simulink model "double_pendulum_2"  (R2022a)
settings: Solver=FixedStepAuto  StartTime=0.0  StopTime=100  FixedStep=0.001  RelTol=1e-3
libraries: sm_lib x8, fl_lib x8, nesl_utility x8, simulink x6
settings Model: Creator=keonyoung  LastModifiedBy=keonyoung

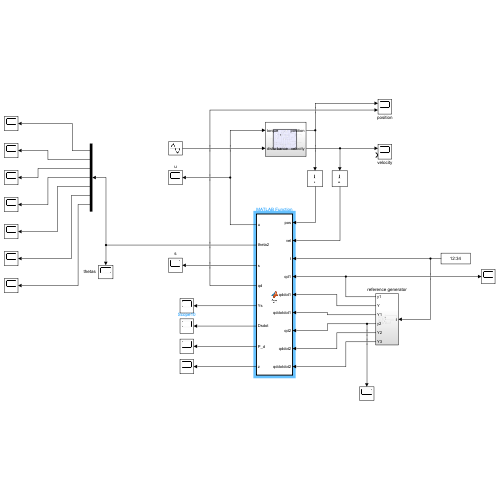
[thumbnail: Simulink's stored preview of the top-level diagram]
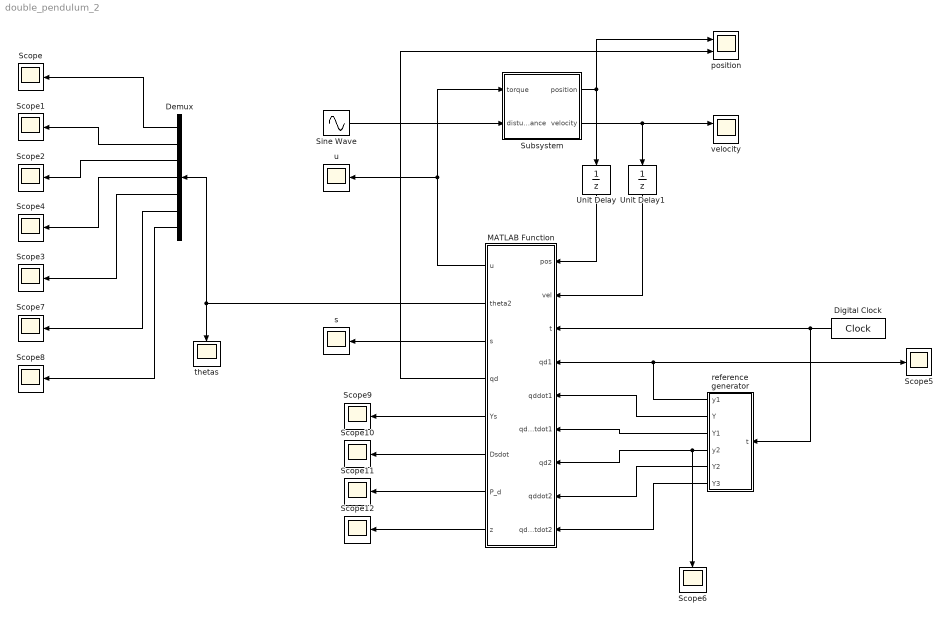
== system double_pendulum_2 ==
  Demux : Demux  Outputs=7
  Digital Clock : DigitalClock  SampleTime=0.001
  MATLAB Function : MATLAB Function  TreatAsAtomicUnit=on
  Scope{,1..12} (13 alike) : Scope
  Sine Wave : Sin  Amplitude=0  SampleTime=0
  Subsystem : Subsystem
  Unit Delay : UnitDelay  SampleTime=-1  HasFrameUpgradeWarning=on
  Unit Delay1 : UnitDelay  SampleTime=-1  HasFrameUpgradeWarning=on
  position : Scope  NumInputPorts=2
  reference generator : Subsystem
  s : Scope
  thetas : Scope
  u : Scope
  velocity : Scope  NumInputPorts=2
  wires:
  MATLAB Function/1(u) -> Subsystem/1(torque), u/1
  Sine Wave/1 -> Subsystem/2(disturbance)
  Subsystem/1(position) -> position/1, Unit Delay/1
  Subsystem/2(velocity) -> Unit Delay1/1, velocity/1
  Digital Clock/1 -> MATLAB Function/3(t), reference generator/1(t)
  Unit Delay/1 -> MATLAB Function/1(pos)
  Unit Delay1/1 -> MATLAB Function/2(vel)
  MATLAB Function/2(theta2) -> Demux/1, thetas/1
  MATLAB Function/3(s) -> s/1
  MATLAB Function/4(qd) -> position/2
  Demux/3 -> Scope2/1
  Demux/4 -> Scope4/1
  Demux/5 -> Scope3/1
  Demux/2 -> Scope1/1
  Demux/1 -> Scope/1
  reference generator/1(y1) -> Scope5/1, MATLAB Function/4(qd1)
  reference generator/2(Y) -> MATLAB Function/5(qddot1)
  reference generator/3(Y1) -> MATLAB Function/6(qddotdot1)
  reference generator/4(y2) -> Scope6/1, MATLAB Function/7(qd2)
  reference generator/5(Y2) -> MATLAB Function/8(qddot2)
  reference generator/6(Y3) -> MATLAB Function/9(qddotdot2)
  Demux/6 -> Scope7/1
  Demux/7 -> Scope8/1
  MATLAB Function/5(Ys) -> Scope9/1
  MATLAB Function/6(Dsdot) -> Scope10/1
  MATLAB Function/7(P_d) -> Scope11/1
  MATLAB Function/8(z) -> Scope12/1

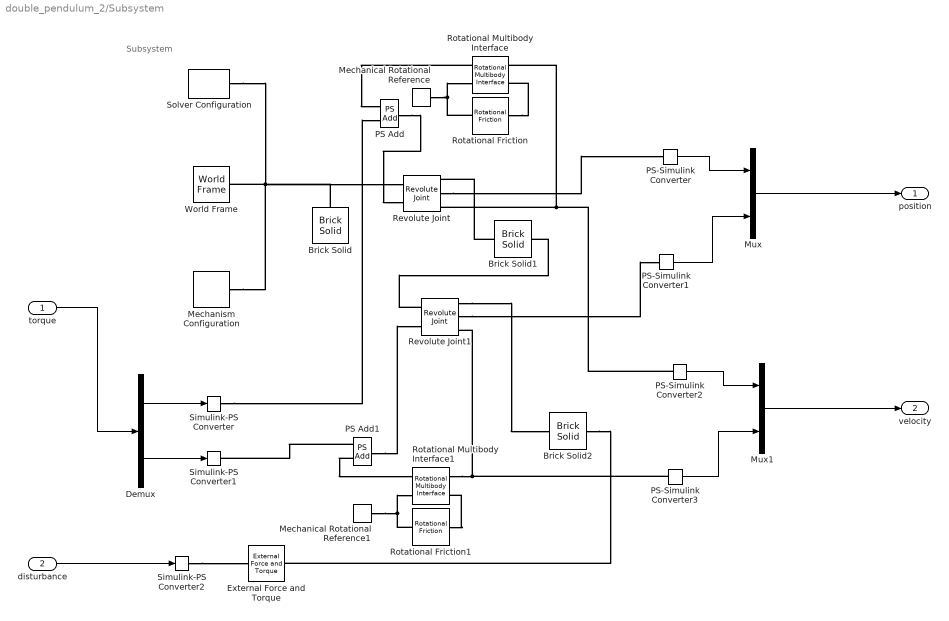
== system double_pendulum_2/Subsystem ==
  note: Subsystem
  torque : Inport
  disturbance : Inport  Port=2
  Brick Solid : sm_lib/Body Elements/Brick Solid  GraphicAmbientColor=[0.15 0.15 0.15 1.0]  BasedOnType=Density  BrickDimensions=[1 0.1 0.1]  BrickDimensionUnits=m  CenterOfMass=[0 0 0]  CenterOfMassUnits=m  GraphicDiffuseColor=[0.5 0.5 0.5]  Density=1000  DensityUnits=kg/m^3  DoExposeReferenceFrame=on  GraphicEmissiveColor=[0.0 0.0 0.0 1.0]  ExportEntireGeometry=off  SerializedFrames=<Frames/>  MarkerShape=Sphere  MarkerSize=10  GraphicType=FromGeometry  InertiaType=CalculateFromGeometry  Mass=1  MassUnits=kg  MomentsOfInertia=[1 1 1]  MomentsOfInertiaUnits=kg*m^2  GraphicOpacity=1.0  ProductsOfInertia=[0 0 0]  ProductsOfInertiaUnits=kg*m^2  GraphicShininess=75  GraphicSpecularColor=[0.5 0.5 0.5 1.0]  GraphicVisPropType=SimpleVisualProperties
  Brick Solid1 : sm_lib/Body Elements/Brick Solid  GraphicAmbientColor=[0.15 0.15 0.15 1.0]  BasedOnType=Mass  BrickDimensions=[0.269 0.04 0.02]  BrickDimensionUnits=m  CenterOfMass=[0 0 0]  CenterOfMassUnits=m  GraphicDiffuseColor=[0.0 0.2 0.8]  Density=7800  DensityUnits=kg/m^3  DoExposeReferenceFrame=off  GraphicEmissiveColor=[0.0 0.0 0.0 1.0]  ExportEntireGeometry=off  SerializedFrames=<Frames><Frame><Id>Frame1</Id><Value><Name>F1</Name><Origin><Source>GeometricFeature</Source><FeatureName>-x surface</FeatureName></Origin><PrimaryAxis><DefinedDirection>+Z</DefinedDirection><Source>ReferenceFrame</Source><SourceDirection>+Z</SourceDirection><FeatureName></FeatureName></PrimaryAxis><SecondaryAxis><DefinedDirection>+X</DefinedDirection><Source>ReferenceFrame</Source><SourceDirection>+X</SourceDirection><FeatureName></FeatureName></SecondaryAxis></Value></Frame><Frame><Id>Frame2</Id><Value><Name>F2</Name><Origin><Source>GeometricFeature</Source><FeatureName>+x surface</FeatureName></Origin><PrimaryAxis><DefinedDirection>+Z</DefinedDirection><Source>ReferenceFrame</Source><SourceDirection>+Z</SourceDirection><FeatureName></FeatureName></PrimaryAxis><SecondaryAxis><DefinedDirection>+X</DefinedDirection><Source>ReferenceFrame</Source><SourceDirection>+X</SourceDirection><FeatureName></FeatureName></SecondaryAxis></Value></Frame></Frames>  MarkerShape=Sphere  MarkerSize=10  GraphicType=FromGeometry  InertiaType=CalculateFromGeometry  Mass=1.75  MassUnits=kg  MomentsOfInertia=[1 1 1]  MomentsOfInertiaUnits=kg*m^2  GraphicOpacity=1.0  ProductsOfInertia=[0 0 0]  ProductsOfInertiaUnits=kg*m^2  GraphicShininess=75  GraphicSpecularColor=[0.5 0.5 0.5 1.0]  GraphicVisPropType=SimpleVisualProperties
  Brick Solid2 : sm_lib/Body Elements/Brick Solid  GraphicAmbientColor=[0.15 0.15 0.15 1.0]  BasedOnType=Mass  BrickDimensions=[0.343 0.04 0.02]  BrickDimensionUnits=m  CenterOfMass=[0 0 0]  CenterOfMassUnits=m  GraphicDiffuseColor=[0.8 0.0 0.4]  Density=7800  DensityUnits=kg/m^3  DoExposeReferenceFrame=off  GraphicEmissiveColor=[0.0 0.0 0.0 1.0]  ExportEntireGeometry=off  SerializedFrames=<Frames><Frame><Id>Frame1</Id><Value><Name>F1</Name><Origin><Source>GeometricFeature</Source><FeatureName>-x surface</FeatureName></Origin><PrimaryAxis><DefinedDirection>+Z</DefinedDirection><Source>ReferenceFrame</Source><SourceDirection>+Z</SourceDirection><FeatureName></FeatureName></PrimaryAxis><SecondaryAxis><DefinedDirection>+X</DefinedDirection><Source>ReferenceFrame</Source><SourceDirection>+X</SourceDirection><FeatureName></FeatureName></SecondaryAxis></Value></Frame><Frame><Id>Frame2</Id><Value><Name>F2</Name><Origin><Source>GeometricFeature</Source><FeatureName>+x surface</FeatureName></Origin><PrimaryAxis><DefinedDirection>+Z</DefinedDirection><Source>ReferenceFrame</Source><SourceDirection>+Z</SourceDirection><FeatureName></FeatureName></PrimaryAxis><SecondaryAxis><DefinedDirection>+X</DefinedDirection><Source>ReferenceFrame</Source><SourceDirection>+X</SourceDirection><FeatureName></FeatureName></SecondaryAxis></Value></Frame></Frames>  MarkerShape=Sphere  MarkerSize=10  GraphicType=FromGeometry  InertiaType=CalculateFromGeometry  Mass=1.89  MassUnits=kg  MomentsOfInertia=[1 1 1]  MomentsOfInertiaUnits=kg*m^2  GraphicOpacity=1.0  ProductsOfInertia=[0 0 0]  ProductsOfInertiaUnits=kg*m^2  GraphicShininess=75  GraphicSpecularColor=[0.5 0.5 0.5 1.0]  GraphicVisPropType=SimpleVisualProperties
  Demux : Demux  Outputs=2
  External Force and Torque : sm_lib/Forces and Torques/External Force and Torque  ForceResolutionFrame=AttachedFrame  EnableForceX=on  EnableForceY=off  EnableForceZ=off  EnableForce=off  TorqueResolutionFrame=AttachedFrame  EnableTorqueX=off  EnableTorqueY=off  EnableTorqueZ=off  EnableTorque=off
  Mechanical Rotational Reference : fl_lib/Mechanical/Rotational Elements/Mechanical Rotational Reference
      settings: SourceProductBaseCode=PW,SS,VE
  Mechanical Rotational Reference1 : fl_lib/Mechanical/Rotational Elements/Mechanical Rotational Reference
      settings: SourceProductBaseCode=PW,SS,VE
  Mechanism Configuration : sm_lib/Utilities/Mechanism Configuration  UniformGravity=Constant  GravityVector=[0 -9.80665 0]  GravityUnits=m/s^2  LinearizationDelta=0.001  JointModeTransitionNonlinearIterations=2
  Mux : Mux  Inputs=2
  Mux1 : Mux  Inputs=2
  PS Add : fl_lib/Physical Signals/Functions/PS Add
      settings: SourceProductBaseCode=PW,SS,VE
  PS Add1 : fl_lib/Physical Signals/Functions/PS Add
      settings: SourceProductBaseCode=PW,SS,VE
  PS-Simulink Converter : nesl_utility/PS-Simulink Converter  PhysicalDomain=network_engine_domain  SubClassName=ps_output  LeftPortType=input  RightPortType=output  PseudoPeriodic=off  Frequencies=[]  VectorFormat=inherit  Unit=rad  AffineConversion=off
      settings: SourceProductBaseCode=SS,PW,VE
  PS-Simulink Converter1 : nesl_utility/PS-Simulink Converter  PhysicalDomain=network_engine_domain  SubClassName=ps_output  LeftPortType=input  RightPortType=output  PseudoPeriodic=off  Frequencies=[]  VectorFormat=inherit  Unit=rad  AffineConversion=off
      settings: SourceProductBaseCode=SS,PW,VE
  PS-Simulink Converter2 : nesl_utility/PS-Simulink Converter  PhysicalDomain=network_engine_domain  SubClassName=ps_output  LeftPortType=input  RightPortType=output  PseudoPeriodic=off  Frequencies=[]  VectorFormat=inherit  Unit=rad/s  AffineConversion=off
      settings: SourceProductBaseCode=SS,PW,VE
  PS-Simulink Converter3 : nesl_utility/PS-Simulink Converter  PhysicalDomain=network_engine_domain  SubClassName=ps_output  LeftPortType=input  RightPortType=output  PseudoPeriodic=off  Frequencies=[]  VectorFormat=inherit  Unit=rad/s  AffineConversion=off
      settings: SourceProductBaseCode=SS,PW,VE
  Revolute Joint : sm_lib/Joints/Revolute Joint  JointMode=Normal  SenseConstraintForce=off  SenseConstraintForceX=off  SenseConstraintForceY=off  SenseConstraintForceZ=off  SenseConstraintTorque=off  SenseConstraintTorqueX=off  SenseConstraintTorqueY=off  SenseConstraintTorqueZ=off  SenseTotalForce=off  SenseTotalForceX=off  SenseTotalForceY=off  SenseTotalForceZ=off  SenseTotalTorque=off  SenseTotalTorqueX=off  SenseTotalTorqueY=off  SenseTotalTorqueZ=off  CompositeWrenchDir=FollowerOnBase  CompositeWrenchFrame=BaseFrame  EquilibriumPosition=0  EquilibriumPositionUnits=deg  SpringStiffness=0  SpringStiffnessUnits=N*m/deg  DampingCoefficient=0  DampingCoefficientUnits=N*m/(rad/s)  TorqueActuationMode=InputTorque  MotionActuationMode=ComputedMotion  SensePosition=on  SenseVelocity=on  SenseAcceleration=off  SenseTorqueForce=off  SenseLowerLimitTorqueForce=off  SenseUpperLimitTorqueForce=off  LowerLimitSpecify=off  LowerLimitBound=-90  LowerLimitBoundUnits=deg  LowerLimitStiffness=1e4  LowerLimitStiffnessUnits=N*m/deg  LowerLimitDamping=10  LowerLimitDampingUnits=N*m/(deg/s)  LowerLimitTransitionRegionWidth=0.1  LowerLimitTransitionRegionWidthUnits=deg  UpperLimitSpecify=off  UpperLimitBound=90  UpperLimitBoundUnits=deg  UpperLimitStiffness=1e4  UpperLimitStiffnessUnits=N*m/deg  UpperLimitDamping=10  UpperLimitDampingUnits=N*m/(deg/s)  UpperLimitTransitionRegionWidth=0.1  UpperLimitTransitionRegionWidthUnits=deg  PositionTargetSpecify=on  PositionTargetPriority=High  PositionTargetValue=-pi/2  PositionTargetValueUnits=rad  VelocityTargetSpecify=off  VelocityTargetPriority=High  VelocityTargetValue=0  VelocityTargetValueUnits=rad/s
  Revolute Joint1 : sm_lib/Joints/Revolute Joint  JointMode=Normal  SenseConstraintForce=off  SenseConstraintForceX=off  SenseConstraintForceY=off  SenseConstraintForceZ=off  SenseConstraintTorque=off  SenseConstraintTorqueX=off  SenseConstraintTorqueY=off  SenseConstraintTorqueZ=off  SenseTotalForce=off  SenseTotalForceX=off  SenseTotalForceY=off  SenseTotalForceZ=off  SenseTotalTorque=off  SenseTotalTorqueX=off  SenseTotalTorqueY=off  SenseTotalTorqueZ=off  CompositeWrenchDir=FollowerOnBase  CompositeWrenchFrame=BaseFrame  EquilibriumPosition=0  EquilibriumPositionUnits=deg  SpringStiffness=0  SpringStiffnessUnits=N*m/deg  DampingCoefficient=0  DampingCoefficientUnits=N*m/(deg/s)  TorqueActuationMode=InputTorque  MotionActuationMode=ComputedMotion  SensePosition=on  SenseVelocity=on  SenseAcceleration=off  SenseTorqueForce=off  SenseLowerLimitTorqueForce=off  SenseUpperLimitTorqueForce=off  LowerLimitSpecify=off  LowerLimitBound=-90  LowerLimitBoundUnits=deg  LowerLimitStiffness=1e4  LowerLimitStiffnessUnits=N*m/deg  LowerLimitDamping=10  LowerLimitDampingUnits=N*m/(deg/s)  LowerLimitTransitionRegionWidth=0.1  LowerLimitTransitionRegionWidthUnits=deg  UpperLimitSpecify=off  UpperLimitBound=90  UpperLimitBoundUnits=deg  UpperLimitStiffness=1e4  UpperLimitStiffnessUnits=N*m/deg  UpperLimitDamping=10  UpperLimitDampingUnits=N*m/(deg/s)  UpperLimitTransitionRegionWidth=0.1  UpperLimitTransitionRegionWidthUnits=deg  PositionTargetSpecify=off  PositionTargetPriority=High  PositionTargetValue=0  PositionTargetValueUnits=deg  VelocityTargetSpecify=off  VelocityTargetPriority=High  VelocityTargetValue=0  VelocityTargetValueUnits=rad/s
  Rotational Friction : fl_lib/Mechanical/Rotational Elements/Rotational Friction  brkwy_trq=2 N*m  brkwy_vel=0.001 rad/s  Col_trq=2 N*m  visc_coef=0.5 N*m*s/rad  w_specify=off  w_priority=None  w=0 rad/s  w_nominal_specify=off  w_nominal_unit=rad/s  w_nominal_value=1  t_specify=off  t_priority=None  t=0 N*m  t_nominal_specify=off  t_nominal_unit=N*m  t_nominal_value=1
      settings: SourceProductBaseCode=PW,SS,VE
  Rotational Friction1 : fl_lib/Mechanical/Rotational Elements/Rotational Friction  brkwy_trq=2 N*m  brkwy_vel=0.001 rad/s  Col_trq=2 N*m  visc_coef=0.5 N*m*s/rad  w_specify=off  w_priority=None  w=0 rad/s  w_nominal_specify=off  w_nominal_unit=rad/s  w_nominal_value=1  t_specify=off  t_priority=None  t=0 N*m  t_nominal_specify=off  t_nominal_unit=N*m  t_nominal_value=1
      settings: SourceProductBaseCode=PW,SS,VE
  Rotational Multibody Interface : fl_lib/Mechanical/Multibody Interfaces/Rotational Multibody Interface
      settings: SourceProductBaseCode=PW,SS,VE
  Rotational Multibody Interface1 : fl_lib/Mechanical/Multibody Interfaces/Rotational Multibody Interface
      settings: SourceProductBaseCode=PW,SS,VE
  Simulink-PS Converter : nesl_utility/Simulink-PS Converter  PhysicalDomain=network_engine_domain  SubClassName=ps_input  LeftPortType=input  RightPortType=output  PseudoPeriodic=off  Frequencies=[]  NoiseDistribution=none  NoiseParameters=[]  Unit=N*m  AffineConversion=off  FilteringAndDerivatives=provide  SimscapeFilterOrder=1  InputFilterTimeConstant=0.001  UdotUserProvided=0
      settings: SourceProductBaseCode=SS,PW,VE
  Simulink-PS Converter1 : nesl_utility/Simulink-PS Converter  PhysicalDomain=network_engine_domain  SubClassName=ps_input  LeftPortType=input  RightPortType=output  PseudoPeriodic=off  Frequencies=[]  NoiseDistribution=none  NoiseParameters=[]  Unit=N*m  AffineConversion=off  FilteringAndDerivatives=provide  SimscapeFilterOrder=1  InputFilterTimeConstant=0.001  UdotUserProvided=0
      settings: SourceProductBaseCode=SS,PW,VE
  Simulink-PS Converter2 : nesl_utility/Simulink-PS Converter  PhysicalDomain=network_engine_domain  SubClassName=ps_input  LeftPortType=input  RightPortType=output  PseudoPeriodic=off  Frequencies=[]  NoiseDistribution=none  NoiseParameters=[]  Unit=1  AffineConversion=off  FilteringAndDerivatives=provide  SimscapeFilterOrder=1  InputFilterTimeConstant=0.001  UdotUserProvided=0
      settings: SourceProductBaseCode=SS,PW,VE
  Solver Configuration : nesl_utility/Solver Configuration  PhysicalDomain=network_engine_domain  SubClassName=solver  LeftPortType=input  RightPortType=generic  Tones=[]  Harmonics=[]  SimulateNoise=off  Profile=off  UseLocalSampling=off  EnableSwitchedLinearOptims=on  FrequencyDomain=off  UseCCode=off  RelTol=0.001  AbsTol=0.001  MinStep=1e-09  ToWorkspace=off  RevertToSquareIcSolve=off  NumHomotopyIterations=100  PhasorMode=off  PhasorModeNumHarmonics=1  IndexReductionMethod=DerivativeReplacement  DoDC=off  ResidualTolerance=1e-09  UseLocalSolver=off  LocalSolverChoice=NE_BACKWARD_EULER_ADVANCER  LocalSolverSampleTime=0.001  DoFixedCost=off  MaxNonlinIter=3  MaxModeIter=2  ComputeImpulses=off  ImpulseIterations=2  LinearAlgebra=auto  LinearAlgebraNumThread=0  EquationFormulation=NE_TIME_EF  DelaysMemoryBudget=1024  AutomaticFiltering=on  FilteringTimeConstant=0.001  PartitionStorageMethod=AS_NEEDED  PartitionMemoryBudget=1024  PartitionMethod=ROBUST
      settings: SourceProductBaseCode=SS,PW,VE
  World Frame : sm_lib/Frames and Transforms/World Frame
  position : Outport
  velocity : Outport  Port=2
  wires:
  Demux/2 -> Simulink-PS Converter1/1
  PS-Simulink Converter/1 -> Mux/1
  Demux/1 -> Simulink-PS Converter/1
  PS-Simulink Converter3/1 -> Mux1/2
  PS-Simulink Converter1/1 -> Mux/2
  PS-Simulink Converter2/1 -> Mux1/1
  Mux1/1 -> velocity/1
  Mux/1 -> position/1
  torque/1 -> Demux/1
  disturbance/1 -> Simulink-PS Converter2/1
  connections:
  Brick Solid2/RConn1 -- External Force and Torque/RConn1
  Mechanism Configuration/RConn1 -- Brick Solid/RConn1 -- Revolute Joint/LConn1 -- World Frame/RConn1 -- Solver Configuration/RConn1
  Revolute Joint1/RConn2 -- PS-Simulink Converter1/LConn1
  Simulink-PS Converter2/RConn1 -- External Force and Torque/LConn1
  Revolute Joint1/RConn1 -- Brick Solid2/LConn1
  PS-Simulink Converter2/LConn1 -- Revolute Joint/RConn3 -- Rotational Multibody Interface/RConn1
  PS-Simulink Converter3/LConn1 -- Revolute Joint1/RConn3 -- Rotational Multibody Interface1/RConn1
  Revolute Joint/RConn2 -- PS-Simulink Converter/LConn1
  Revolute Joint1/LConn1 -- Brick Solid1/RConn1
  Brick Solid1/LConn1 -- Revolute Joint/RConn1
  Rotational Friction/LConn1 -- Rotational Multibody Interface/RConn2
  Rotational Friction/RConn1 -- Rotational Multibody Interface/LConn2 -- Mechanical Rotational Reference/LConn1
  Simulink-PS Converter/RConn1 -- PS Add/LConn2
  Rotational Multibody Interface/LConn1 -- PS Add/LConn1
  PS Add/RConn1 -- Revolute Joint/LConn2
  Rotational Friction1/LConn1 -- Rotational Multibody Interface1/RConn2
  Rotational Friction1/RConn1 -- Rotational Multibody Interface1/LConn2 -- Mechanical Rotational Reference1/LConn1
  PS Add1/LConn1 -- Simulink-PS Converter1/RConn1
  PS Add1/LConn2 -- Rotational Multibody Interface1/LConn1
  PS Add1/RConn1 -- Revolute Joint1/LConn2

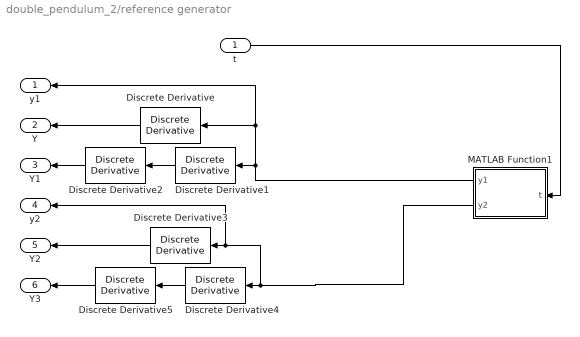
== system double_pendulum_2/reference generator ==
  t : Inport
  Discrete Derivative{,1..5} (6 alike) : simulink/Discrete/Discrete Derivative  gainval=1.0  ICPrevScaledInput=0.0  OutMin=[]  OutMax=[]  OutDataType=fixdt(1, 16)  OutScaling=2^-10  DoSatur=off
  MATLAB Function1 : MATLAB Function  TreatAsAtomicUnit=on
  y1 : Outport
  Y : Outport  Port=2
  Y1 : Outport  Port=3
  y2 : Outport  Port=4
  Y2 : Outport  Port=5
  Y3 : Outport  Port=6
  wires:
  Discrete Derivative2/1 -> Y1/1
  MATLAB Function1/1(y1) -> y1/1, Discrete Derivative/1, Discrete Derivative1/1
  t/1 -> MATLAB Function1/1(t)
  Discrete Derivative1/1 -> Discrete Derivative2/1
  Discrete Derivative4/1 -> Discrete Derivative5/1
  MATLAB Function1/2(y2) -> y2/1, Discrete Derivative3/1, Discrete Derivative4/1
  Discrete Derivative/1 -> Y/1
  Discrete Derivative3/1 -> Y2/1
  Discrete Derivative5/1 -> Y3/1

== matlab function double_pendulum_2/reference generator/MATLAB Function1 ==
  data: t input; y1 output; y2 output
function [y1, y2]= fcn(t)

% ver 1 %%
% persistent ti1;
% persistent yi1;
% persistent tf1;
% persistent yf1;
% persistent T1;
% persistent flag1;
% persistent count1;
% persistent ti2;
% persistent yi2;
% persistent tf2;
% persistent yf2;
% persistent T2;
% persistent flag2;
% persistent count2;
% 
% if isempty(ti1)
%     ti1 = 0;
%     yi1 = 0;
%     tf1 = rand + 1;
%     yf1 = pi/6*rand + pi/6;
%     T1 = tf1-ti1;
%     flag1 = 0;
%     count1 = 0;
%     ti2 = 0;
%     yi2 = 0;
%     tf2 = rand + 1;
%     yf2 = pi/6*rand + pi/6;
%     T2 = tf1-ti1;
%     flag2 = 0;
%     count2 = 0;
% end
% 
% x1 = t-count1;
% x2 = t-count2;
% 
% if flag1 == 0
%     a = (yf1-yi1)/2;
%     y1 = a*sin(2*pi/(2*T1)*(x1-T1/2))+a+yi1;
% else
%     a = -(yf1-yi1)/2;
%     y1 = a*sin(2*pi/(2*T1)*(x1+T1/2))+yi1-a;
% end
% 
% if flag2 == 0
%     a = (yf2-yi2)/2;
%     y2 = a*sin(2*pi/(2*T2)*(x2-T2/2))+a+yi2;
% else
%     a = -(yf2-yi2)/2;
%     y2 = a*sin(2*pi/(2*T2)*(x2+T2/2))+yi2-a;
% end
% 
% if x1 >= T1
%     count1 = count1 + T1;
%     if flag1 == 0
%         ti1 = tf1;
%         yi1 = yf1;
%         tf1 = rand + 1 + count1;
%         yf1 = -pi/6*rand - pi/6;
%         T1 = tf1 - ti1;
%         flag1 = 1;
%     else
%         ti1 = tf1;
%         yi1 = yf1;
%         tf1 = rand + 1 + count1;
%         yf1 = pi/6*rand + pi/6;
%         T1 = tf1 - ti1;
%         flag1 = 0;
%     end
% end
% 
% if x2 >= T2
%     count2 = count2 + T2;
%     if flag2 == 0
%         ti2 = tf2;
%         yi2 = yf2;
%         tf2 = rand + 1 + count2;
%         yf2 = -pi/6*rand - pi/6;
%         T2 = tf2 - ti2;
%         flag2 = 1;
%     else
%         ti2 = tf2;
%         yi2 = yf2;
%         tf2 = rand + 1 + count2;
%         yf2 = pi/6*rand + pi/6;
%         T2 = tf2 - ti2;
%         flag2 = 0;
%     end
% end


%% ver 2 %%

global_T1 = 0.5*rand + 0.5;
global_T2 = 0.5*rand + 0.5;

persistent ti1;
persistent yi1;
persistent tf1;
persistent yf1;
persistent T1;
persistent flag1;
persistent count1;
persistent ti2;
persistent yi2;
persistent tf2;
persistent yf2;
persistent T2;
persistent flag2;
persistent count2;

if isempty(ti1)
    ti1 = 0;
    yi1 = 0;
    tf1 = global_T1;
    yf1 = pi/6*rand + pi/6;
    T1 = tf1-ti1;
    flag1 = 0;
    count1 = 0;
    ti2 = 0;
    yi2 = 0;
    tf2 = global_T2;
    yf2 = pi/6*rand + pi/6;
    T2 = tf1-ti1;
    flag2 = 0;
    count2 = 0;
end

x1 = t-count1;
x2 = t-count2;

if flag1 == 0
    a = (yf1-yi1)/2;
    y1 = a*sin(2*pi/(2*T1)*(x1-T1/2))+a+yi1;
else
    a = -(yf1-yi1)/2;
    y1 = a*sin(2*pi/(2*T1)*(x1+T1/2))+yi1-a;
end

if flag2 == 0
    a = (yf2-yi2)/2;
    y2 = a*sin(2*pi/(2*T2)*(x2-T2/2))+a+yi2;
else
    a = -(yf2-yi2)/2;
    y2 = a*sin(2*pi/(2*T2)*(x2+T2/2))+yi2-a;
end

if x1 >= T1
    count1 = count1 + T1;
    if flag1 == 0
        ti1 = tf1;
        yi1 = yf1;
        tf1 = global_T1 + count1;
        yf1 = -pi/6*rand - pi/6;
        T1 = tf1 - ti1;
        flag1 = 1;
    else
        ti1 = tf1;
        yi1 = yf1;
        tf1 = global_T1 + count1;
        yf1 = pi/6*rand + pi/6;
        T1 = tf1 - ti1;
        flag1 = 0;
    end
end

if x2 >= T2
    count2 = count2 + T2;
    if flag2 == 0
        ti2 = tf2;
        yi2 = yf2;
        tf2 = global_T2 + count2;
        yf2 = -pi/6*rand - pi/6;
        T2 = tf2 - ti2;
        flag2 = 1;
    else
        ti2 = tf2;
        yi2 = yf2;
        tf2 = global_T2 + count2;
        yf2 = pi/6*rand + pi/6;
        T2 = tf2 - ti2;
        flag2 = 0;
    end
end


%% ver 3

% a1 = pi/3;
% a2 = pi/4;
% w1 = pi/4;
% w2 = pi/4;
% y1 = a1*sin(w1*t)-w1*a1*t-pi/2
% y2 = a2*sin(w2*t)-w2*a2*t;

== matlab function double_pendulum_2/MATLAB Function ==
  data: pos input; u output; vel input; t input; theta2 output; s output; qd output; qd1 input; qddot1 input; qddotdot1 input; qd2 input; qddot2 input; qddotdot2 input; Ys output; Dsdot output; P_d output; z output
function [u, theta2, s, qd, Ys, Dsdot, P_d, z]= fcn(pos, vel, t, qd1, qddot1, qddotdot1, qd2, qddot2, qddotdot2)

persistent theta;
persistent t_theta;
persistent velpast;
persistent P;
persistent spast;
    
g = 9.80665;
lambda = 10; % originally 10
gamma = [1 0.1 0.05 1 1 10 5]'*0.1;
K = 10; % originally 6

t_m1 = 1.75;
t_m2 = 1.89;
l1 = 0.269;
lc1 = 0.1345;
l2 = 0.343;
lc2 = 0.1715;
m1 = l1*0.04*0.02*7800;
m2 = l2*0.04*0.02*7800;
I1 = 1/12*(4*l1^2+0.04^2)*m1;
I2 = 1/12*(4*l2^2+0.04^2)*m2;
t_I1 = 1/12*(4*l1^2+0.04^2)*t_m1;
t_I2 = 1/12*(4*l2^2+0.04^2)*t_m2;

if isempty(theta)
    theta = [m1*lc1^2+m2*(l1^2+lc2^2)+I1+I2; m2*lc2^2+I2; m2*l1*lc2; m1*lc1+m2*l1; m2*lc2; 1; 1];
    t_theta = [t_m1*lc1^2+t_m2*(l1^2+lc2^2)+t_I1+t_I2; t_m2*lc2^2+t_I2; t_m2*l1*lc2; t_m1*lc1+t_m2*l1; t_m2*lc2;2;0.5]
    velpast = [0;0];
    P = diag([1 1 1 1 1 1 1])*0.1;
    spast = [0;0];
end

q1 = pos(1);
q2 = pos(2);
q1dot = vel(1);
q2dot = vel(2);
qd1 = qd1 - pi/2;

% w1 = pi;
% w2 = pi/3;
% a1 = pi/4;
% a2 = pi/2;
% qd = [a1*sin(w1*t)-pi/2; a2*sin(w2*t)];
% qddot = [a1*w1*cos(w1*t); a2*w2*cos(w2*t)];
% qddotdot = [-a1*w1^2*sin(w1*t); -a2*w2^2*sin(w2*t)];
% qd = [t-pi/2;t];
% qddot = [1;1];
% qddotdot = [0;0];

% x = t-count;
% if x >= 9
%     count = count + 9;
% end
% qd = [x^4*(x-1)*(x-3)*(x-5)*(x-7)*(x-9)^4/1000000-pi/2;0];
% qddot = [((-9+x)^3*x^3*(-945 + 2190*x-1557*x^2+467*x^3-62*x^4+3*x^5))/250000;0];
% qddotdot = [((-9 + x)^2 *x^2* (25515 - 84510* x + 85395* x^2 - 37674* x^3 + 8109* x^4 - 836* x^5 + 33* x^6))/250000;0];

qd = [qd1; qd2];
qddot = [qddot1; qddot2];
qddotdot = [qddotdot1; qddotdot2];

s = vel-qddot + lambda*(pos-qd);
z = qddotdot - lambda*(vel-qddot);

%% Tracking-error based estimation
y11 = z(1);
y12 = z(2);
y13 = (2*z(1)+z(2))*cos(q2)-(2*q1dot*q2dot+q2dot^2)*sin(q2);
y14 = g*cos(q1);
y15 = g*cos(q1+q2);
y16 = tanh(20*q1dot);
y17 = q1dot;

y21 = 0;
y22 = z(1)+z(2);
y23 = z(1)*cos(q2)+q1dot^2*sin(q2);
y24 = 0;
y25 = g*cos(q1+q2);
y26 = tanh(20*q2dot);
y27 = q2dot;

Y = [y11, y12, y13, y14, y15, y16, y17; y21, y22, y23, y24, y25, y26, y27];
% Y = [z(1), z(2), (2*z(1) + z(2))*cos(q2) - (2*q1dot*q2dot + q1dot^2)*sin(q2), g*cos(q1), g*cos(q1 + q2);
%         0, z(1) + z(2), z(1)*cos(q2) + (q1dot^2)*sin(q2), 0, g*cos(q1 + q2)];
% theta2 = (theta - t_theta)./t_theta * 100;
% theta = theta - gamma.*transpose(Y)*s*0.001;

% s_bound = 0.5;
% 
% if abs(s(1)) > s_bound
%     sat_s1 = sign(s(1));
% else
%     sat_s1 = s(1)/s_bound;
% end
% 
% if abs(s(2)) > s_bound
%     sat_s2 = sign(s(2));
% else
%     sat_s2 = s(2)/s_bound;
% end


s_bound = 0.5; % originally 0.5

if abs(s(1)) > s_bound
    s(1) = sign(s(1))*s_bound;
else
    s(1) = s(1);
end

if abs(s(2)) > s_bound
    s(2) = sign(s(2))*s_bound;
else
    s(2) = s(2);
end

Ys = gamma.*transpose(Y)*s;

%% prediction-error based estimation
d11 = theta(1) + theta(3)*cos(q2);
d12 = theta(2) + theta(3)*cos(q2);
d21 = theta(2) + theta(3)*cos(q2);
d22 = theta(2);
P = P - P*transpose(Y)*Y*P*0.001;
P_d = diag(transpose(P)*P);
D = [d11 d12; d21 d22];

sdot = (vel-velpast)/0.001 - qddotdot + lambda*(vel - qddot);
% sdot = (s-spast)/0.001;

e = D*sdot + K*s;
Dsdot = transpose(Y)*e;
velpast = vel;
% P_d = 1;
% Dsdot = 1;

%% control law
theta = theta - gamma.*transpose(Y)*s*0.001;
theta = theta - P*transpose(Y)*e*0.001;
theta2 = (theta - t_theta)./t_theta * 100;

u = Y*theta - K*s;
spast = s;
